simulink model "ChildrenModel"  (R2022a)
settings: Solver=VariableStepAuto  StartTime=0.0  StopTime=100  RelTol=1e-3
values from neighbouring files (symbols this model uses):
  delay = Patient(patient,11)    [LoadPatient.m]
  E0 = Patient(patient,9)    [LoadPatient.m]
  E50 = Patient(patient,13)    [LoadPatient.m]
  gamma = Patient(patient,14)    [LoadPatient.m]
  k = Patient(patient,12)    [LoadPatient.m]
  peak = 500    [CalculaModelo.m]
settings Model: Creator=mluser  LastModifiedBy=phcs

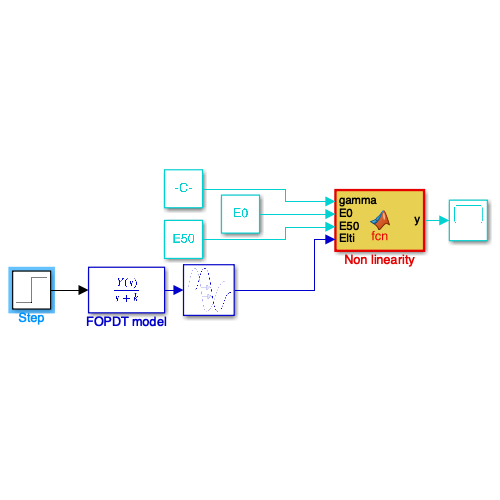
[thumbnail: Simulink's stored preview of the top-level diagram]
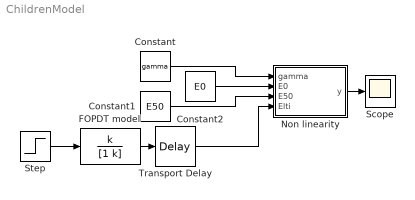
== system ChildrenModel ==
  Constant : Constant  Value=gamma
  Constant1 : Constant  Value=E50
  Constant2 : Constant  Value=E0
  FOPDT model : TransferFcn  Numerator=k  Denominator=[1 k]
  Non linearity : MATLAB Function  TreatAsAtomicUnit=on
  Scope : Scope
  Step : Step  After=peak  SampleTime=0
  Transport Delay : TransportDelay  DelayTime=delay/60
  wires:
  FOPDT model/1 -> Transport Delay/1
  Step/1 -> FOPDT model/1
  Non linearity/1(y) -> Scope/1
  Constant2/1 -> Non linearity/2(E0)
  Constant1/1 -> Non linearity/3(E50)
  Constant/1 -> Non linearity/1(gamma)
  Transport Delay/1 -> Non linearity/4(Elti)

== matlab function ChildrenModel/Non linearity ==
  data: gamma input; y output; E0 input; E50 input; Elti input
function y = fcn(gamma,E0,E50,Elti)

y = E0-E0*Elti^gamma/(E50^gamma+Elti^gamma);
